simulink model "Copy_of_IpSDKSebesegEsPozicio"  (R2013b)
settings: Solver=FixedStepDiscrete  SolverMode=SingleTasking  StartTime=0.0  StopTime=10.0  FixedStep=1  RelTol=1e-3
undefined symbols (not defined in the file or in its folder): gcbh, xlBlockLoadCallback, xlGetNormalizedPeriod
libraries: xbsIndex_r4 x218
(part 1 of 3)
settings Model: Creator=laca  LastModifiedBy=laca
settings DebuggingCC: MultiTaskDSMMsg=warning  MultiTaskCondExecSysMsg=none  FcnCallInpInsideContextMsg=EnableAllAsWarning
settings RTWCC: IncludeERTFirstTime=on

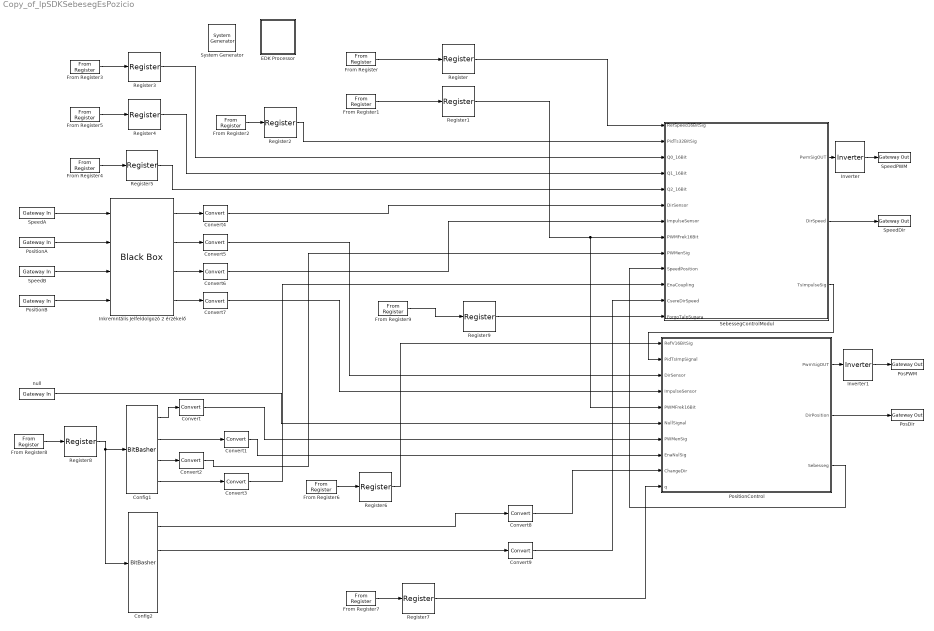
== system Copy_of_IpSDKSebesegEsPozicio ==
  " System Generator" : xbsIndex_r4/ System Generator  Tag=genX  xilinxfamily=spartan3e  part=xc3s500e  speed=-4  package=pq208  synthesis_tool=XST  clock_wrapper=Clock Enables  directory=./netlist  proj_type=Project Navigator  Synth_file=XST Defaults  Impl_file=ISE Defaults  testbench=off  simulink_period=1  sysclk_period=10  dcm_input_clock_period=10  incr_netlist=off  trim_vbits=Everywhere in SubSystem  dbl_ovrd=According to Block Masks  core_generation=According to Block Masks  run_coregen=off  deprecated_control=off  eval_field=0  block_type=sysgen
  Config1 : xbsIndex_r4/BitBasher  bitexpr=|  display_expr=off  sr_1=1  arith_type1=Unsigned  bin_pt1=0  sr_2=2  arith_type2=Unsigned  bin_pt2=0  sr_3=3  arith_type3=Unsigned  bin_pt3=0  sr_4=4  arith_type4=Unsigned  bin_pt4=0  dbl_ovrd=off  block_type=bitbasher
      | <!DOCTYPE HTML PUBLIC "-//W3C//DTD HTML 4.0//EN" "http://www.w3.org/TR/REC-html40/strict.dtd">
      | <html><head><meta name="qrichtext" content="1" /><style type="text/css">
      | p, li { white-space: pre-wrap; }
      | </style></head><body style=" font-family:'MS Shell Dlg 2'; font-size:8.25pt; font-weight:400; font-style:normal;">
      | <p style=" margin-top:12px; margin-bottom:12px; margin-left:0px; margin-right:0px; -qt-block-indent:0; text-indent:0px;"><span style=" font-family:'MS Shell Dlg'; font-size:8pt;">a0={a[0]}<br /></span><span style=" font-family:'MS Shell Dlg'; font-size:8pt;">a1={a[1]}<br />a2={a[2]}<br />a3={a[3]}</span></p></body></html>
  Config2 : xbsIndex_r4/BitBasher  bitexpr=|  display_expr=off  sr_1=1  arith_type1=Unsigned  bin_pt1=0  sr_2=2  arith_type2=Unsigned  bin_pt2=0  sr_3=3  arith_type3=Unsigned  bin_pt3=0  sr_4=4  arith_type4=Unsigned  bin_pt4=0  dbl_ovrd=off  block_type=bitbasher
      | <!DOCTYPE HTML PUBLIC "-//W3C//DTD HTML 4.0//EN" "http://www.w3.org/TR/REC-html40/strict.dtd">
      | <html><head><meta name="qrichtext" content="1" /><style type="text/css">
      | p, li { white-space: pre-wrap; }
      | </style></head><body style=" font-family:'MS Shell Dlg 2'; font-size:8.25pt; font-weight:400; font-style:normal;">
      | <p style=" margin-top:12px; margin-bottom:12px; margin-left:0px; margin-right:0px; -qt-block-indent:0; text-indent:0px;"><span style=" font-family:'MS Shell Dlg'; font-size:8pt;">a4={a[4]}<br />a5={a[5]}<br />a6={a[6]}<br />a7={a[7]}</span></p></body></html>
  Convert{,1..9} (10 alike) : xbsIndex_r4/Convert  gui_display_data_type=Boolean  arith_type=Boolean  n_bits=16  bin_pt=14  float_type=Single  exp_bits=8  fraction_bits=24  quantization=Truncate  overflow=Wrap  en=off  latency=0  dbl_ovrd=off  pipeline=off  block_type=convert
  EDK Processor : Subsystem  LoadFcn=xlBlockLoadCallback(gcbh);  mask(Xilinx EDK Processor Block){mode=EDK pcore generation, xmp=, MemVisToProc=<qt bgcolor="#FFFFFF"><div><img src="C:/Xilinx/14.7/ISE_DS/ISE/sysgen/data/images/registerminus.gif"> &lt;&lt;Config&gt;&gt;<br> <img src="C:/Xilinx/14.7/ISE_DS/ISE/sysgen/data/images/parameters.gif"> Type : Fix_16_0<br> <img src="C:/Xilinx/14.7/ISE_DS/ISE/sysgen/data/images/parameters.gif"> Addr : 0x80000800<br></div><div><img src="C:/Xilinx/14.7/ISE_DS/ISE/sysgen/data/images/registerplus.gif"> &lt;&lt;PosRef&gt;&gt;<br></div><div><img src="C:/Xilinx/14.7/ISE_DS/ISE/sysgen/data/images/registerplus.gif"> &lt;&lt;Q1&gt;&gt;<br></div><div><img src="C:/Xilinx/14.7/ISE_DS/ISE/sysgen/data/images/registerplus.gif"> &lt;&lt;Q2&gt;&gt;<br></div><div><img src="C:/Xilinx/14.7/ISE_DS/ISE/sysgen/data/images/registerplus.gif"> &lt;&lt;Q0&gt;&gt;<br></div><div><img src="C:/Xilinx/14.7/ISE_DS/ISE/sysgen/data/images/registerplus.gif"> &lt;&lt;PidTs&gt;&gt;<br></div><div><img src="C:/Xilinx/14.7/ISE_DS/ISE/sysgen/data/images/registerplus.gif"> &lt;&lt;PWMfrek&gt;&gt;<br></div><div><img src="C:/Xilinx/14.7/ISE_DS/ISE/sysgen/data/images/registerminus.gif"> &lt;&lt;RefSpeed&gt;&gt;<br> <img src="C:/Xilinx/14.7/ISE_DS/ISE/sysgen/data/images/parameters.gif"> Type : Fix_16_0<br> <img src="C:/Xilinx/14.7/ISE_DS/ISE/sysgen/data/images/parameters.gif"> Addr : 0x8000081C<br></div><div><img src="C:/Xilinx/14.7/ISE_DS/ISE/sysgen/data/images/registerplus.gif"> &lt;&lt;SugarakAranya&gt;&gt;<br></div><div><img src="C:/Xilinx/14.7/ISE_DS/ISE/sysgen/data/images/registerplus.gif"> &lt;&lt;q_sav&gt;&gt;<br></div><div><img src="C:/Xilinx/14.7/ISE_DS/ISE/sysgen/data/images/registerminus.gif"> &lt;&lt;USebesseg&gt;&gt;<br> <img src="C:/Xilinx/14.7/ISE_DS/ISE/sysgen/data/images/parameters.gif"> Type : Fix_32_0<br> <img src="C:/Xilinx/14.7/ISE_DS/ISE/sysgen/data/images/parameters.gif"> Addr : 0x80000800<br></div><div><img src="C:/Xilinx/14.7/ISE_DS/ISE/sysgen/data/images/registerplus.gif"> &lt;&lt;UPozicio&gt;&gt;<br></div><div><img src="C:/Xilinx/14.7/ISE_DS/ISE/sysgen/data/images/registerplus.gif"> &lt;&lt;SebessegPozicio&gt;&gt;<br></div><div><img src="C:/Xilinx/14.7/ISE_DS/ISE/sysgen/data/images/registerplus.gif"> &lt;&lt;AktPozicio&gt;&gt;<br></div><div><img src="C:/Xilinx/14.7/ISE_DS/ISE/sysgen/data/images/registerminus.gif"> &lt;&lt;AktSebesseg&gt;&gt;<br> <img src="C:/Xilinx/14.7/ISE_DS/ISE/sysgen/data/images/parameters.gif"> Type : Fix_16_0<br> <img src="C:/Xilinx/14.7/ISE_DS/ISE/sysgen/data/images/parameters.gif"> Addr : 0x80000810<br></div><div><img src="C:/Xilinx/14.7/ISE_DS/ISE/sysgen/data/images/registerplus.gif"> &lt;&lt;eSebesseg&gt;&gt;<br></div></qt>, AvailableMemories=<empty>, portInterfaceTable={'exposed'=>[],'portdir'=>[],'portname'=>[],'shortname'=>[]}, bus_type_sgadvanced=, bus_type=PLB, baseaddr=0x80000000, baseaddr_lock_sgadvanced=, baseaddr_lock=off, dual_clock_sgadvanced=, dual_clock=off, reg_readback_sgadvanced=, reg_readback=off, ucf_file=, inheritDeviceType_sgadvanced=, inheritDeviceType=off, elf_file=, codebug_sgadvanced=, codebug=on, clock_name=plb, internalPortList={}, resetPolarity=0, memxtable={'mladdr'=>[0.00000000000000000,1.00000000000000000,2.00000000000000000,3.00000000000000000,4.00000000000000000,5.00000000000000000,6.00000000000000000,7.00000000000000000,8.00000000000000000,9.00000000000000000,0.00000000000000000,1.00000000000000000,2.00000000000000000,3.00000000000000000,4.00000000000000000,5.00000000000000000],'mlist'=>['IpSDKSebesegEsPozicio/From Register8','IpSDKSebesegEsPozicio/From Register6','IpSDKSebesegEsPozicio/From Register5','IpSDKSebesegEsPozicio/From Register4','IpSDKSebesegEsPozicio/From Register3','IpSDKSebesegEsPozicio/From Register2','IpSDKSebesegEsPozicio/From Register1','IpSDKSebesegEsPozicio/From Register','IpSDKSebesegEsPozicio/From Register9','IpSDKSebesegEsPozicio/From Register7','IpSDKSebesegEsPozicio/SebessegControlModul/To Register2','IpSDKSebesegEsPozicio/PositionControl/To Register3','IpSDKSebesegEsPozicio/PositionControl/To Register2','IpSDKSebesegEsPozicio/PositionControl/To Register1','IpSDKSebesegEsPozicio/SebessegControlModul/To Register1','IpSDKSebesegEsPozicio/SebessegControlModul/To Register3'],'mlname'=>['\'Config\'','\'PosRef\'','\'Q1\'','\'Q2\'','\'Q0\'','\'PidTs\'','\'PWMfrek\'','\'RefSpeed\'','\'SugarakAranya\'','\'q_sav\'','\'USebesseg\'','\'UPozicio\'','\'SebessegPozicio\'','\'AktPozicio\'','\'AktSebesseg\'','\'eSebesseg\''],'mlstate'=>[1.00000000000000000,0.00000000000000000,0.00000000000000000,0.00000000000000000,0.00000000000000000,0.00000000000000000,0.00000000000000000,1.00000000000000000,0.00000000000000000,0.00000000000000000,1.00000000000000000,0.00000000000000000,0.00000000000000000,0.00000000000000000,1.00000000000000000,0.00000000000000000]}, procinfo={}, memmapdirty=off, blockname=, xpsintstyle=default, has_advanced_control=0, sggui_pos=2162,313,385,441, block_type=edkprocessor, block_version=2.7, sg_icon_stat=62,63,-1,-1,white,blue,0,07734,right,,[ ],[ ], sg_mask_display=|, sg_list_contents={'table'=>{'AvailableMemories'=>'popup(<empty>)'}}, sg_blockgui_xml=}
      mask sg_mask_display=|
      | fprintf('','COMMENT: begin icon graphics');
      | patch([0 62 62 0 0 ],[0 0 63 63 0 ],[0.77 0.82 0.91 ]);
      | plot([0 62 62 0 0 ],[0 0 63 63 0 ]);
      | patch([13.2 24.76 32.76 40.76 48.76 32.76 21.2 13.2 ],[39.88 39.88 47.88 39.88 47.88 47.88 47.88 39.88 ],[1 1 1 ]);
      | patch([21.2 32.76 24.76 13.2 21.2 ],[31.88 31.88 39.88 39.88 31.88 ],[0.931 0.946 0.973 ]);
      | patch([13.2 24.76 32.76 21.2 13.2 ],[23.88 23.88 31.88 31.88 23.88 ],[1 1 1 ]);
      | patch([21.2 48.76 40.76 32.76 24.76 13.2 21.2 ],[15.88 15.88 23.88 15.88 23.88 23.88 15.88 ],[0.931 0.946 0.973 ]);
      | fprintf('','COMMENT: end icon graphics');
      | fprintf('','COMMENT: begin icon text');
      | fprintf('','COMMENT: end icon text');
      mask prompts: mode "Configure Processor for"; xmp "XPS Project"; MemVisToProc ""; AvailableMemories "Available Memories"; portInterfaceTable ""; bus_type_sgadvanced ""; bus_type "Bus Type"; baseaddr "Base Address"; baseaddr_lock_sgadvanced ""; baseaddr_lock "Lock"; dual_clock_sgadvanced ""; dual_clock "Dual Clocks"; reg_readback_sgadvanced ""; reg_readback "Register Read-Back"; ucf_file "Constraint File"; inheritDeviceType_sgadvanced ""; inheritDeviceType "Inherit Device Type"; elf_file "Initial Program"; codebug_sgadvanced ""; codebug "Enable Co-Debug with Xilinx SDK (Beta)"; clock_name ""; internalPortList ""; resetPolarity ""; memxtable ""; procinfo ""; memmapdirty ""; blockname ""; xpsintstyle ""; has_advanced_control ""; sggui_pos ""; block_type ""; block_version ""; sg_icon_stat ""; sg_mask_display ""; sg_list_contents ""; sg_blockgui_xml ""
      mask help: Xilinx EDK Processor
      mask init:
      | try
      |   tmp_gcb = gcb;
      |   tmp_gcbh = gcbh;
      |   if (strcmp('SysGenIndex',get_param(bdroot(tmp_gcbh),'tag')) && ~isempty(regexp(bdroot(tmp_gcb), '^xbs', 'once')))
      |     return;
      |   end;
      |   xlMungeMaskParams;
      | 
      |   block_type='edkprocessor';
      | 
      |   serialized_declarations = '{''block_type''=>''String''}';
      |   xledkprocessor_init();
      |   ptable_ = xlblockprep(get_param(tmp_gcb, 'MaskWSVariables'));
      |   try
      |     xlBlockMoveCallback(tmp_gcbh);
      |   catch 
      |      clear global xl_updateicon_recursion_guard;
      |   end;
      | catch
      |   global dbgsysgen;
      |   if(~isempty(dbgsysgen) && dbgsysgen)
      |     e = regexprep(lasterr, '\n', '\nError: ');
      |     disp(['Error: While running MaskInit code on block ' tmp_gcb ': ' e]);
      |     error(e);
      |   end
      | end
      settings: CopyFcn=xlProcBlockCopyCallback(gcbh);xlBlockMoveCallback(gcbh);  DeleteFcn=xlDestroyGui(gcbh);  ModelCloseFcn=xlDestroyGui(gcbh);  PreSaveFcn=xlBlockPreSaveCallback(gcbh);  PostSaveFcn=xlBlockPostSaveCallback(gcbh);  DestroyFcn=xlDestroyGui(gcbh);  OpenFcn=bh=gcbh;xlProcBlockCallbacks('populatesharedmemorylistbox',bh);xlOpenGui(bh, 'edkprocessor_gui.xml', @xlProcBlockEnablement, @xlProcBlockAction);  CloseFcn=xlDestroyGui(gcbh);  MoveFcn=xlBlockMoveCallback(gcbh);
      mask Help: eval('');xlDoc('-book','sysgen','-topic','EDK_Processor');
      mask TypeOptions mode: EDK pcore generation | HDL netlisting
      mask TypeOptions bus_type: AXI | PLB
      mask Display:
      | fprintf('','COMMENT: begin icon graphics');
      | patch([0 62 62 0 0 ],[0 0 63 63 0 ],[0.77 0.82 0.91 ]);
      | plot([0 62 62 0 0 ],[0 0 63 63 0 ]);
      | patch([13.2 24.76 32.76 40.76 48.76 32.76 21.2 13.2 ],[39.88 39.88 47.88 39.88 47.88 47.88 47.88 39.88 ],[1 1 1 ]);
      | patch([21.2 32.76 24.76 13.2 21.2 ],[31.88 31.88 39.88 39.88 31.88 ],[0.931 0.946 0.973 ]);
      | patch([13.2 24.76 32.76 21.2 13.2 ],[23.88 23.88 31.88 31.88 23.88 ],[1 1 1 ]);
      | patch([21.2 48.76 40.76 32.76 24.76 13.2 21.2 ],[15.88 15.88 23.88 15.88 23.88 23.88 15.88 ],[0.931 0.946 0.973 ]);
      | fprintf('','COMMENT: end icon graphics');
      | fprintf('','COMMENT: begin icon text');
      | disp('');
      | 
      | fprintf('','COMMENT: end icon text');
  From Register : xbsIndex_r4/From Register  shared_memory_name='RefSpeed'  init=0  period=1  ownership=Locally owned and initialized  gui_display_data_type=Fixed-point  arith_type="Signed  (2's comp)"  n_bits=16  bin_pt=0  preci_type=Single  dbl_ovrd=off  block_type=fromreg
      settings: AttributesFormatString=<< %<shared_memory_name> >>  infoedit="Register block that reads data to a shared memory register.  Delay of one sample period."
  From Register1 : xbsIndex_r4/From Register  shared_memory_name='PWMfrek'  init=0  period=1  ownership=Locally owned and initialized  gui_display_data_type=Fixed-point  arith_type=Unsigned  n_bits=16  bin_pt=0  preci_type=Single  dbl_ovrd=off  block_type=fromreg
      settings: AttributesFormatString=<< %<shared_memory_name> >>  infoedit="Register block that reads data to a shared memory register.  Delay of one sample period."
  From Register2 : xbsIndex_r4/From Register  shared_memory_name='PidTs'  init=0  period=1  ownership=Locally owned and initialized  gui_display_data_type=Fixed-point  arith_type=Unsigned  n_bits=32  bin_pt=0  preci_type=Single  dbl_ovrd=off  block_type=fromreg
      settings: AttributesFormatString=<< %<shared_memory_name> >>  infoedit="Register block that reads data to a shared memory register.  Delay of one sample period."
  From Register3 : xbsIndex_r4/From Register  shared_memory_name='Q0'  init=0  period=1  ownership=Locally owned and initialized  gui_display_data_type=Fixed-point  arith_type="Signed  (2's comp)"  n_bits=16  bin_pt=0  preci_type=Single  dbl_ovrd=off  block_type=fromreg
      settings: AttributesFormatString=<< %<shared_memory_name> >>  infoedit="Register block that reads data to a shared memory register.  Delay of one sample period."
  From Register4 : xbsIndex_r4/From Register  shared_memory_name='Q2'  init=0  period=1  ownership=Locally owned and initialized  gui_display_data_type=Fixed-point  arith_type=Unsigned  n_bits=16  bin_pt=0  preci_type=Single  dbl_ovrd=off  block_type=fromreg
      settings: AttributesFormatString=<< %<shared_memory_name> >>  infoedit="Register block that reads data to a shared memory register.  Delay of one sample period."
  From Register5 : xbsIndex_r4/From Register  shared_memory_name='Q1'  init=0  period=1  ownership=Locally owned and initialized  gui_display_data_type=Fixed-point  arith_type="Signed  (2's comp)"  n_bits=16  bin_pt=0  preci_type=Single  dbl_ovrd=off  block_type=fromreg
      settings: AttributesFormatString=<< %<shared_memory_name> >>  infoedit="Register block that reads data to a shared memory register.  Delay of one sample period."
  From Register6 : xbsIndex_r4/From Register  shared_memory_name='PosRef'  init=0  period=1  ownership=Locally owned and initialized  gui_display_data_type=Fixed-point  arith_type="Signed  (2's comp)"  n_bits=16  bin_pt=0  preci_type=Single  dbl_ovrd=off  block_type=fromreg
      settings: AttributesFormatString=<< %<shared_memory_name> >>  infoedit="Register block that reads data to a shared memory register.  Delay of one sample period."
  From Register7 : xbsIndex_r4/From Register  shared_memory_name='q_sav'  init=0  period=1  ownership=Locally owned and initialized  gui_display_data_type=Fixed-point  arith_type=Unsigned  n_bits=16  bin_pt=0  preci_type=Single  dbl_ovrd=off  block_type=fromreg
      settings: AttributesFormatString=<< %<shared_memory_name> >>  infoedit="Register block that reads data to a shared memory register.  Delay of one sample period."
  From Register8 : xbsIndex_r4/From Register  shared_memory_name='Config'  init=0  period=1  ownership=Locally owned and initialized  gui_display_data_type=Fixed-point  arith_type=Unsigned  n_bits=16  bin_pt=0  preci_type=Single  dbl_ovrd=off  block_type=fromreg
      settings: AttributesFormatString=<< %<shared_memory_name> >>  infoedit="Register block that reads data to a shared memory register.  Delay of one sample period."
  From Register9 : xbsIndex_r4/From Register  shared_memory_name='SugarakAranya'  init=0  period=1  ownership=Locally owned and initialized  gui_display_data_type=Fixed-point  arith_type="Signed  (2's comp)"  n_bits=16  bin_pt=0  preci_type=Single  dbl_ovrd=off  block_type=fromreg
      settings: AttributesFormatString=<< %<shared_memory_name> >>  infoedit="Register block that reads data to a shared memory register.  Delay of one sample period."
  Inkremntális Jelfeldolgozó 2 érzékelő : xbsIndex_r4/Black Box  init_code=SensorIncModul2Sensor_config  sim_method=ISE Simulator  verbose=off  block_type=blackbox2
      settings: xl_use_area=on  xl_area=[100,0,0,0,0,0,0]
  Inverter : xbsIndex_r4/Inverter  en=off  latency=0  dbl_ovrd=off  block_type=inv
  Inverter1 : xbsIndex_r4/Inverter  en=off  latency=0  dbl_ovrd=off  block_type=inv
  PosDir : xbsIndex_r4/Gateway Out  inherit_from_input=off  hdl_port=on  timing_constraint=None  locs_specified=off  LOCs={}  UseAsDAC=off  DACChannel='1'  block_type=gatewayout
      settings: xl_area=[0 0 0 0 1 0 0]
  PosPWM : xbsIndex_r4/Gateway Out  inherit_from_input=off  hdl_port=on  timing_constraint=None  locs_specified=off  LOCs={}  UseAsDAC=off  DACChannel='1'  block_type=gatewayout
      settings: xl_area=[0 0 0 0 1 0 0]
  PositionA : xbsIndex_r4/Gateway In  gui_display_data_type=Boolean  arith_type=Boolean  n_bits=16  bin_pt=14  preci_type=Single  exp_width=8  frac_width=24  quantization="Round  (unbiased: +/- Inf)"  overflow=Saturate  period=1  dbl_ovrd=off  timing_constraint=None  locs_specified=off  LOCs={}  UseAsADC=off  ADCChannel='1'  inherit_from_input=off  hdl_port=on  block_type=gatewayin
      settings: xl_area=[0 0 0 0 1 0 0]
  PositionB : xbsIndex_r4/Gateway In  gui_display_data_type=Boolean  arith_type=Boolean  n_bits=16  bin_pt=14  preci_type=Single  exp_width=8  frac_width=24  quantization="Round  (unbiased: +/- Inf)"  overflow=Saturate  period=1  dbl_ovrd=off  timing_constraint=None  locs_specified=off  LOCs={}  UseAsADC=off  ADCChannel='1'  inherit_from_input=off  hdl_port=on  block_type=gatewayin
      settings: xl_area=[0 0 0 0 1 0 0]
  PositionControl : Subsystem
  Register{,1..9} (10 alike) : xbsIndex_r4/Register  init=0  rst=off  en=off  dbl_ovrd=off  block_type=register
      Register2 settings: xl_use_area=on  xl_area=[100,0,0,0,0,0,0]
      Register6 settings: xl_use_area=on  xl_area=[100,0,0,0,0,0,0]
      Register9 settings: xl_use_area=on  xl_area=[100,0,0,0,0,0,0]
  SebessegControlModul : Subsystem
  SpeedA : xbsIndex_r4/Gateway In  gui_display_data_type=Boolean  arith_type=Boolean  n_bits=16  bin_pt=14  preci_type=Single  exp_width=8  frac_width=24  quantization="Round  (unbiased: +/- Inf)"  overflow=Saturate  period=1  dbl_ovrd=off  timing_constraint=None  locs_specified=off  LOCs={}  UseAsADC=off  ADCChannel='1'  inherit_from_input=off  hdl_port=on  block_type=gatewayin
      settings: xl_area=[0 0 0 0 1 0 0]
  SpeedB : xbsIndex_r4/Gateway In  gui_display_data_type=Boolean  arith_type=Boolean  n_bits=16  bin_pt=14  preci_type=Single  exp_width=8  frac_width=24  quantization="Round  (unbiased: +/- Inf)"  overflow=Saturate  period=1  dbl_ovrd=off  timing_constraint=None  locs_specified=off  LOCs={}  UseAsADC=off  ADCChannel='1'  inherit_from_input=off  hdl_port=on  block_type=gatewayin
      settings: xl_area=[0 0 0 0 1 0 0]
  SpeedDir : xbsIndex_r4/Gateway Out  inherit_from_input=off  hdl_port=on  timing_constraint=None  locs_specified=off  LOCs={}  UseAsDAC=off  DACChannel='1'  block_type=gatewayout
      settings: xl_area=[0 0 0 0 1 0 0]
  SpeedPWM : xbsIndex_r4/Gateway Out  inherit_from_input=off  hdl_port=on  timing_constraint=None  locs_specified=off  LOCs={}  UseAsDAC=off  DACChannel='1'  block_type=gatewayout
      settings: xl_area=[0 0 0 0 1 0 0]
  null : xbsIndex_r4/Gateway In  gui_display_data_type=Fixed-point  arith_type=Unsigned  n_bits=1  bin_pt=0  preci_type=Single  exp_width=8  frac_width=24  quantization="Round  (unbiased: +/- Inf)"  overflow=Saturate  period=1  dbl_ovrd=off  timing_constraint=None  locs_specified=off  LOCs={}  UseAsADC=off  ADCChannel='1'  inherit_from_input=off  hdl_port=on  block_type=gatewayin
      settings: xl_area=[0 0 0 0 1 0 0]
  wires:
  From Register1/1 -> Register1/1
  From Register3/1 -> Register3/1
  From Register4/1 -> Register5/1
  Config1/3 -> Convert2/1
  Config1/1 -> Convert/1
  SebessegControlModul/3(TsImpulseSig) -> PositionControl/2(PidTsImpSignal)
  From Register6/1 -> Register6/1
  null/1 -> PositionControl/6(NullSignal)
  PositionControl/3(Sebesseg) -> SebessegControlModul/10(SpeedPosition)
  Config1/4 -> Convert3/1
  Config1/2 -> Convert1/1
  SebessegControlModul/2(DirSpeed) -> SpeedDir/1
  PositionControl/2(DirPosition) -> PosDir/1
  From Register2/1 -> Register2/1
  From Register5/1 -> Register4/1
  From Register8/1 -> Register8/1
  Convert/1 -> PositionControl/7(PWMenSig)
  Convert1/1 -> PositionControl/8(EnaNulSig)
  Convert2/1 -> SebessegControlModul/9(PWMenSig)
  Convert3/1 -> SebessegControlModul/11(EnaCoupling)
  Convert4/1 -> SebessegControlModul/6(DirSensor)
  Convert5/1 -> PositionControl/3(DirSensor)
  Convert6/1 -> SebessegControlModul/7(ImpulseSensor)
  Convert7/1 -> PositionControl/4(ImpulseSensor)
  Inkremntális Jelfeldolgozó 2 érzékelő/1 -> Convert4/1
  Inkremntális Jelfeldolgozó 2 érzékelő/2 -> Convert5/1
  Inkremntális Jelfeldolgozó 2 érzékelő/3 -> Convert6/1
  Inkremntális Jelfeldolgozó 2 érzékelő/4 -> Convert7/1
  SpeedA/1 -> Inkremntális Jelfeldolgozó 2 érzékelő/1
  PositionA/1 -> Inkremntális Jelfeldolgozó 2 érzékelő/2
  SpeedB/1 -> Inkremntális Jelfeldolgozó 2 érzékelő/3
  PositionB/1 -> Inkremntális Jelfeldolgozó 2 érzékelő/4
  Register/1 -> SebessegControlModul/1(RefSpeed16BitSig)
  Register1/1 -> SebessegControlModul/8(PWMFrek16Bit), PositionControl/5(PWMFrek16Bit)
  Register2/1 -> SebessegControlModul/2(PidTs32BitSig)
  Register3/1 -> SebessegControlModul/3(Q0_16Bit)
  Register4/1 -> SebessegControlModul/4(Q1_16Bit)
  Register5/1 -> SebessegControlModul/5(Q2_16Bit)
  Register6/1 -> PositionControl/1(RefV16BitSig)
  Convert8/1 -> PositionControl/9(ChangeDir)
  Register8/1 -> Config2/1, Config1/1
  Config2/1 -> Convert8/1
  Config2/2 -> Convert9/1
  Convert9/1 -> SebessegControlModul/12(CsereDirSpeed)
  SebessegControlModul/1(PwmSigOUT) -> Inverter/1
  PositionControl/1(PwmSigOUT) -> Inverter1/1
  From Register7/1 -> Register7/1
  Register7/1 -> PositionControl/10(q)
  From Register9/1 -> Register9/1
  Register9/1 -> SebessegControlModul/13(ForgoTalpSugara)
  From Register/1 -> Register/1
  Inverter/1 -> SpeedPWM/1
  Inverter1/1 -> PosPWM/1
